simulink library "cstblocks"  (Simulink 6.0)
settings: Solver=ode45  SolverMode=SingleTasking  StartTime=0.0  StopTime=10.0  RelTol=1e-3
values from neighbouring files (symbols this model uses):
  D = diag(D)    [care.m]    (also in gcare.m = []; gdare.m = [])
undefined symbols (not defined in the file or in its folder): A, B, C, X0
libraries: cstextras x2
settings Model: RequirementInfo=9  ForwardingTableString=||__slOldName__||cstblocks/Input Point||__slNewName__||slctrlobsolete/Input Point||__slOldName__||cstblocks/Output Point||__slNewName__||slctrlobsolete/Output Point  Creator=greg  LastModifiedBy=pascal
settings DataIOCC: SignalLoggingName=logsOut
settings OptimizationCC: BooleanDataType=off
settings DebuggingCC: CheckExecutionContextPreStartOutputMsg=on  CheckExecutionContextRuntimeOutputMsg=on  SolverPrmCheckMsg=none
settings HardwareCC: TargetUnknown=on
settings SFSimCC: SFSimApplyToAllLibs=on  SFSimBuildMode=Incremental

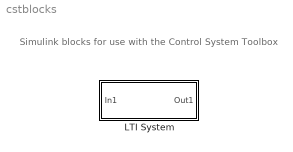
== system cstblocks ==
  note: Simulink blocks for use with the
      | Control System Toolbox
  LTI System : Subsystem  PropExecContextAcrossSSBoundary=on  mask(LTI Block){sys=tf(1,[1 1]), IC=[]}
      mask prompts: sys "LTI system variable"; IC "Initial states   (state-space only)"
      mask help:
      | The LTI System block accepts both continuous and discrete LTI models as defined in the Control System Toolbox. Transfer function, state-space, and zero-pole-gain formats are all supported in this block.
      |
      | Note: Initial states are only meaningful for state-space systems.
      mask init:
      | [A,B,C,D,Ts,Tdi,Tdo,X0,sysname]=ltimask('Initialize',gcb,sys,IC);
      | ltimask('UpdateDiagram',gcb,Ts);
      mask Help:
      | The LTI System block accepts any of the three standard LTI models described in the Control System Toolbox: transfer function, zero/pole/gain, or state space. Internally, LTI models will be converted to their state space equivalent for evaluation.
      | <p>
      | In the editable text box labeled <b>LTI System Variable</b>, enter a valid LTI model.
      | <p>
      | In the editable text box labeled <b>Initial States</b> enter the initial state vector.  Initial states are only valid for state-space systems.
      | <p>
      | See also TF, ZPK, SS, LTIMODELS.
      mask CallbackString: ltimask('MaskLTICallback',gcb);|
      mask Display: disp(sysname)

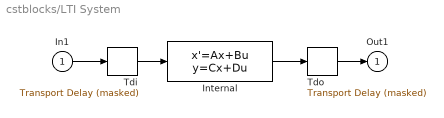
== system cstblocks/LTI System ==
  In1 : Inport  LatchInput=off
  Internal : StateSpace  A=A  B=B  C=C  D=D  X0=X0
  Tdi : cstextras/Transport Delay (masked)  Tag=InputDelayBlock  Td=Tdi  u0=0  bufsize=1024
  Tdo : cstextras/Transport Delay (masked)  Tag=OutputDelayBlock  Td=Tdo  u0=0  bufsize=1024
  Out1 : Outport  InitialOutput=0
  wires:
  In1/1 -> Tdi/1
  Tdi/1 -> Internal/1
  Internal/1 -> Tdo/1
  Tdo/1 -> Out1/1
